simulink model "NonLinearModel"  (Simulink 9.3)
settings: Solver=ode45  StartTime=0.0  StopTime=Tsim  RelTol=1e-10  EnableMultiTasking=on
values from neighbouring files (symbols this model uses):
  alpha_init = 1*x_trim(1)    [FLYmodel.m]
  b = 9.17    [MyAircraft.mat]    (also in longMotion.m = 2.15; trimConfig.m)
  c = 2.15    [MyAircraft.mat]    (also in trimConfig.m)
  CG = 0.245    [MyAircraft.mat]    (also in trimConfig.m)
  el_init = x_trim(2)    [FLYmodel.m]
  eng_init = x_trim(4)    [FLYmodel.m]
  H_init = plane.h    [FLYmodel.m]
  Jgross = [5000 34000 45000 2200]    [MyAircraft.mat]    (also in trimConfig.m = [Ixx Iyy Izz Ixz])
  m = 6500    [MyAircraft.mat]    (also in input_param.m = str2double(answerX{3}); trimConfig.m = plane.m)
  pitch_init = 1*x_trim(3)    [FLYmodel.m]
  plane = input_param    [FLYmodel.m]    (also in MyAircraft.mat = )
  rAC = 0.245    [MyAircraft.mat]    (also in trimConfig.m = plane.x_T)
  rho = 0.823328195592    [MyAircraft.mat]    (also in input_param.m = rho_0*(1-vyska/44308)^4.2553; trimConfig.m = plane.rho)
  S = 18.8    [MyAircraft.mat]    (also in latMotion.m; longMotion.m; trimConfig.m)
  Ts = 1/50    (= 0.02)    [FLYmodel.m]
  v0 = plane.v0    [FLYmodel.m]    (also in MyAircraft.mat = 240; input_param.m = str2double(answerX{1}); trimConfig.m)
  x_trim = trimConfig(plane)    [FLYmodel.m]    (also in MyAircraft.mat = [0 0 0 0]; trimConfig.m = [x(1) x(2) x(3) x(4)])
undefined symbols (not defined in the file or in its folder): Ap, As, Bp, Bs, Cp, Cs, Dp, Ds
undefined symbols (not defined in the file): V_init
libraries: simulink_extras x13
(part 2 of 2)

== matlab function My Aircraft/Aerodynamic model/Embedded MATLAB Function ==
  data: Wind input double; CX output double; Control input double; ABdot input double; AngRates input double; Mach input double; mass input double; CY output double; CZ output double; Cl output double; Cm output double; Cn output double; rho input double; M_const input double
function [CX,CY,CZ,Cl,Cm,Cn] = AeroCoefM(Wind,Control,ABdot,AngRates,Mach,mass,rho,M_const)

V = Wind(1);
beta = Wind(2);
alpha = Wind(3);
de = Control(1);
da = Control(2);
dr = Control(3);
M = Mach;
m = mass;
c = 2.15; % m
S = 18.8; 
b = 9.17;

p = AngRates(1);
q = AngRates(2);
r = AngRates(3);
adot = ABdot(1);
m = mass; 

%% Drag
% Minimum drag
if M<0.4
    CD0 = 0.0223;
elseif M>0.92 
    CD0 = 0.1032;
else
    CD0 = 7.861*M^4 - 18.378*M^3 + 15.832*M^2 - 5.9269*M + 0.8349;
%     CD0 = 7.861*M_const^4 - 18.378*M_const^3 + 15.832*M_const^2 ...
%         - 5.9269*M_const + 0.8349;
end

% alpha derivate
    CDa = 0.00103*(alpha*180/pi)^2 - 0.00308*alpha*180/pi;


% Pitch control (elevator) derivative
CDde = 6.2863E-07*(de*180/pi)^3 + 4.1831E-05*(de*180/pi)^2 -...
    3.1917E-04*(de*180/pi) + 1.6834E-04;


%% Lift
% Zero-alpha lift
    % CL0 = 0.3;
    x_cy0       = [0,0.4,0.6,0.7,0.75,0.8,0.85,0.9]; 
    y_cy0       = [0.09,0.09,0.09,0.105,0.13,0.12,0.07,0.02];
    % pocatecni hodnota vztlakoveho soucinitele
%     CL0 = interp1(x_cy0,y_cy0,M_const);
    CL0 = interp1(x_cy0,y_cy0,M);
    
% alpha derivative
    % CLa = 4.44;
    % derivace soucinitele vztlaku podle uhlu nabehu
    if M <= 0.3
        CLa = 4.4418;
    else
        CLa = - 62.716*M^5 + 122.09*M^4 - 85.797*M^3 + 28.153*M^2 ...
                   - 3.8433*M + 4.541;
    end
% Pitch control (elevator) derivative
    CLde = 0.305;

% alpha-dot derivative
    % CLalphadot = 0;
    % derivace soucinitele vztlaku podle bezrozmerne zmeny uhlu nabehu
    if M<0.3
        Mp = 0.3;
        CLalphadot = -49.167 + 558.542*Mp - 2284.051*Mp^2 ... 
        + 4412.037*Mp^3 - 4067.130*Mp^4 + 1435.185*Mp^5;
    elseif M>0.7
        Mp = 0.7;
        CLalphadot = -49.167 + 558.542*Mp - 2284.051*Mp^2 ... 
        + 4412.037*Mp^3 - 4067.130*Mp^4 + 1435.185*Mp^5;
    else
        CLalphadot = -49.167 + 558.542*M - 2284.051*M^2 ... 
        + 4412.037*M^3 - 4067.130*M^4 + 1435.185*M^5;
    end
% Pitch rate derivative
    % CLq = 3.8;
    % derivace soucinitele vztlaku podle bezrozmerne rychlosti kloneni
%     CLq = 5.7414 - 9.3115*M + 20.8*M^2 - 13.465*M^3;
    tx_M        = [0.0, 0.3, 0.4, 0.5, 0.6, 0.7, 0.75, 0.9];
    tc_y_w      = [4.45, 4.45, 4.5, 4.6, 4.7, 4.85, 4.75, 4.75];
    CLq = interp1(tx_M,tc_y_w,M);


%%% Pitch moment coefficient %%%
% Zero-alpha pitch
    % Cm0 = 0;
    y_mz0 = [0.025,0.025,0.03,0.025,0.02,0.05,-0.02,-0.03];
%     pocatecni hodnota klopiveho soucinitele
%     Cm0 = interp1(x_cy0,y_mz0,M);
    Cm0 = interp1(x_cy0,y_mz0,M_const);
%     Cm0 = 0.025;
% 	if M <= 0.3
%         Cm0 = 0.025;
%     else
%         Cm0 = -0.703*M^3 + 0.828*M^2 - 0.258*M + 0.040;
%     end
    
% alpha derivative
    % Cma = -0.683;
    if M <= 0.3
        Cma = -0.4899;
    else
%         M = M_const;
        Cma = 5.9964*M^4 - 10.271*M^3 + 6.7921*M^2 - 2.0056*M -0.2708;
    end    

% Pitch control derivative
    Cmde = -0.88;
    
% alpha_dot derivative
%     Cmalphadot = -4.36;
    if M <= 0.3
        Cmalphadot = -1.38271969;
    else
        Cmalphadot = 502.427*M^5 - 1303.11*M^4 + 1330.2481*M^3 ...
            - 668.0225*M^2 + 164.08*M - 17.0671;
    end    
% Pitch rate derivative
%     Cmq = -9.96;
    if M <= 0.3
        Cmq = -4.9934668;
    else
        Cmq = 2.5926*M^3 - 8.7063*M^2 + 4.8590*M - 5.7376;
    end    

%% Side force coefficient %%%
    cyPom = m*9.81/(0.5*rho*V^2*S);
    % Sideslip derivative
    % CYbeta = -0.564;
    CYbeta = (-0.946 - 0.0333*cyPom + 0.0032*M - 0.16*M^2);
    % Roll control derivative
    CYda = -0.02;
    % Yaw control derivative
    CYdr = (-0.1845 + 0.0325*cyPom -0.0093*M -0.0228*M^2 ...
        -0.012*M^3);

%% Roll moment coefficient %%%
    % Sideslip derivative
    if M<0.45
        Clbeta = -0.056 - 0.0576*cyPom - 0.0088*M;
    else
        Clbeta = -0.06 - 0.0576*cyPom - 0.0285*(M - 0.45);
    end
    
    % Roll control derivative
    if M<=0.6
        Clda = (-0.156 + 0.04*(M -0.2));
    else
        Clda = -1.1039 + 4.6696*M - 7.5941*M^2 ...
            + 4.1483*M^3;
    end
    
    % Yaw control derivative
    Cldr = (-0.03 + 0.008*cyPom)*1;
    
    % Roll rate derivative
    Clp = -0.5365 - 1.5267*M + 10.781*M^2 ...
        -20.666*M^3 + 12.4242*M^4;
    % Yaw rate derivative
    Clr = (-0.075 - 0.215*cyPom -0.016*M);

%% Yaw moment coefficient %%%
    % Sideslip derivative
    Cnbeta = (-0.173 + 0.01667*cyPom + 0.0092*M -0.1*M^2 +...
        0.0208*M^3);
    
    % Roll control derivative   
    Cnda = -0.0015;
    
    % Yaw control derivative
    Cndr = (0.015*cyPom - 0.095 -0.0056*M -0.0089*M^2 ...
        - 0.0068*M^3);
    
    % Roll rate derivative
    if M<0.7
        Cnp = -0.07435 + 0.045*cyPom - 0.0092*M;
    else
        Cnp = -0.08079 + 0.044*cyPom - 0.0333*(M-0.7);
    end

    % Yaw rate derivative
    Cnr = -0.2291 - 0.0065*cyPom -0.0236*cyPom^2 + 0.0069*cyPom^3 ...
            - 0.0219*M + 0.0097*M^2 - 0.0447*M^3;

CX = CD0 + CDa + CDde;
CY = CYbeta*beta + CYda*da + CYdr*dr;
CZ = CL0 + CLa*alpha + CLde*de + c*q*CLq/V + c*adot*CLalphadot/V;
Cl = Clbeta*beta + b*p*Clp/(2*V) + b*r*Clr/(2*V) + Clda*da + Cldr*dr;
Cm = Cm0 + Cma*alpha + Cmde*de + c*q*Cmq/V + c*adot*Cmalphadot/V;
Cn = Cnbeta*beta + b*p*Cnp/(2*V) + b*r*Cnr/(2*V) + Cnda*da + Cndr*dr;
